simulink model "sysgenMRIDemo"  (Simulink 7.7)
settings: Solver=VariableStepDiscrete  StartTime=0.0  StopTime=inf  RelTol=1e-3
PreLoadFcn:
  | sysgenMRIDemo_PreloadFcn
InitFcn:
  | xlFrameDisplay;
undefined symbols (not defined in the file or in its folder): a, b, c_image_cols, c_image_rows, c_num_fstores, c_swathe_size, sysgenMRIDemo_data_imag_channel, xlFrameDisplay
libraries: xbsIndex_r4 x297, dspsrcs4 x3, xbsCopyrightNotice_r4 x1, simulink x1
(part 2 of 3)

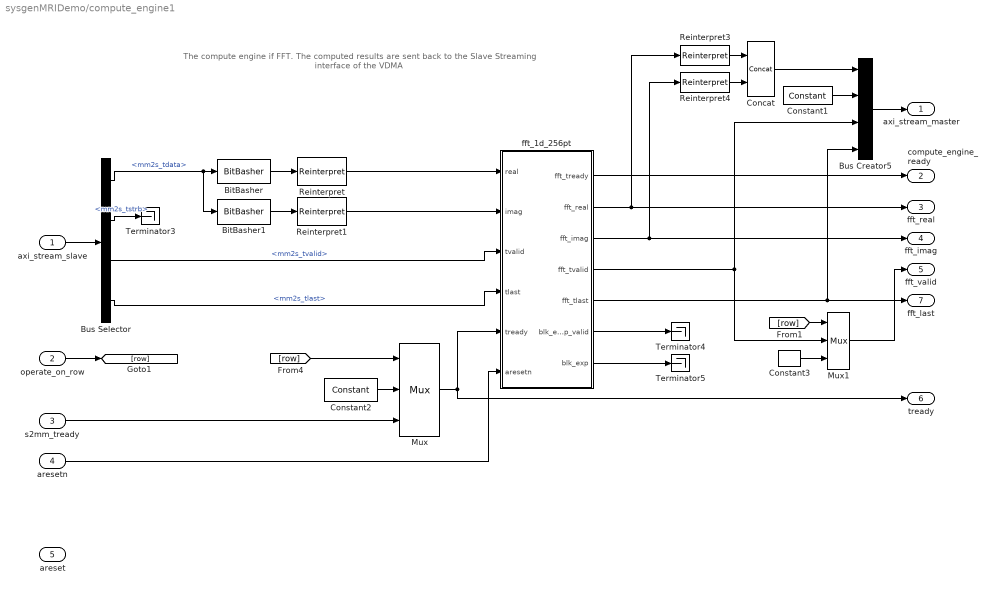
== system sysgenMRIDemo/compute_engine1 ==
  note: The compute engine if FFT. The computed results are sent back
      | to the Slave Streaming interface of the VDMA
  axi_stream_slave : Inport
  operate_on_row : Inport  Port=2
  s2mm_tready : Inport  Port=3
  aresetn : Inport  Port=4
  areset : Inport  Port=5
  BitBasher : xbsIndex_r4/BitBasher  bitexpr=|  display_expr=off  sr_1=1  arith_type1=Unsigned  bin_pt1=0  sr_2=2  arith_type2=Unsigned  bin_pt2=0  sr_3=3  arith_type3=Unsigned  bin_pt3=0  sr_4=4  arith_type4=Unsigned  bin_pt4=0  dbl_ovrd=off  block_type=bitbasher
      | <!DOCTYPE HTML PUBLIC "-//W3C//DTD HTML 4.0//EN" "http://www.w3.org/TR/REC-html40/strict.dtd">
      | <html><head><meta name="qrichtext" content="1" /><style type="text/css">
      | p, li { white-space: pre-wrap; }
      | </style></head><body style=" font-family:'MS Shell Dlg 2'; font-size:7.8pt; font-weight:400; font-style:normal;">
      | <p style=" margin-top:12px; margin-bottom:12px; margin-left:0px; margin-right:0px; -qt-block-indent:0; text-indent:0px;"><span style=" font-family:'MS Shell Dlg'; font-size:8pt;">real = {data[63:32]}</span></p></body></html>
      settings: block_version=12.3
  BitBasher1 : xbsIndex_r4/BitBasher  bitexpr=|  display_expr=off  sr_1=1  arith_type1=Unsigned  bin_pt1=0  sr_2=2  arith_type2=Unsigned  bin_pt2=0  sr_3=3  arith_type3=Unsigned  bin_pt3=0  sr_4=4  arith_type4=Unsigned  bin_pt4=0  dbl_ovrd=off  block_type=bitbasher
      | <!DOCTYPE HTML PUBLIC "-//W3C//DTD HTML 4.0//EN" "http://www.w3.org/TR/REC-html40/strict.dtd">
      | <html><head><meta name="qrichtext" content="1" /><style type="text/css">
      | p, li { white-space: pre-wrap; }
      | </style></head><body style=" font-family:'MS Shell Dlg 2'; font-size:7.8pt; font-weight:400; font-style:normal;">
      | <p style=" margin-top:12px; margin-bottom:12px; margin-left:0px; margin-right:0px; -qt-block-indent:0; text-indent:0px;"><span style=" font-family:'MS Shell Dlg'; font-size:8pt;">imag = {data[31:0]}</span></p></body></html>
      settings: block_version=12.3
  Bus Creator5 : BusCreator
  Bus Selector : BusSelector  OutputSignals=mm2s_tdata,mm2s_tstrb,mm2s_tvalid,mm2s_tlast
  Concat : xbsIndex_r4/Concat  num_inputs=2  dbl_ovrd=off  block_type=concat
      settings: block_version=12.3
  Constant1 : xbsIndex_r4/Constant  const=2^8-1  gui_display_data_type=Fixed-point  arith_type=Unsigned  n_bits=8  bin_pt=0  preci_type=Single  exp_width=8  frac_width=24  explicit_period=on  period=1  equ=P=C  opselect=C  inp2=PCIN>>17  opr=+  inp1=P  carry=CIN  dbl_ovrd=off  block_type=constant
      settings: block_version=12.3
  Constant2 : xbsIndex_r4/Constant  const=1  gui_display_data_type=Fixed-point  arith_type=Boolean  n_bits=8  bin_pt=0  preci_type=Single  exp_width=8  frac_width=24  explicit_period=on  period=1  equ=P=C  opselect=C  inp2=PCIN>>17  opr=+  inp1=P  carry=CIN  dbl_ovrd=off  block_type=constant
      settings: block_version=12.3
  Constant3 : xbsIndex_r4/Constant  const=0  gui_display_data_type=Fixed-point  arith_type=Boolean  n_bits=8  bin_pt=0  preci_type=Single  exp_width=8  frac_width=24  explicit_period=on  period=1  equ=P=C  opselect=C  inp2=PCIN>>17  opr=+  inp1=P  carry=CIN  dbl_ovrd=off  block_type=constant
      settings: block_version=12.3
  Mux : xbsIndex_r4/Mux  inputs=2  en=off  latency=0  precision=Full  arith_type=Unsigned  n_bits=16  bin_pt=14  quantization=Truncate  overflow=Wrap  dbl_ovrd=off  block_type=mux
      settings: block_version=13.0.2
  Mux1 : xbsIndex_r4/Mux  inputs=2  en=off  latency=0  precision=Full  arith_type=Unsigned  n_bits=16  bin_pt=14  quantization=Truncate  overflow=Wrap  dbl_ovrd=off  block_type=mux
      settings: block_version=13.0.2
  Reinterpret : xbsIndex_r4/Reinterpret  force_arith_type=on  arith_type="Signed  (2's comp)"  force_bin_pt=on  bin_pt=31  block_type=reinterpret
      settings: infoedit="Changes signal type without altering the binary representation.   You can changed the signal between signed and unsigned, and relocate the binary point.<br><br>Hardware notes: In hardware this block costs nothing.<br><br>Example:  Suppose the input is 6 bits wide, signed, with 2 fractional bits, and the output is forced to unsigned with 0 fractional bits.  Then an input of -2.0 (1110.00 in binary 2's complement) becomes an output of 56 (111000 in binary)."  block_version=12.3
  Reinterpret1 : xbsIndex_r4/Reinterpret  force_arith_type=on  arith_type="Signed  (2's comp)"  force_bin_pt=on  bin_pt=31  block_type=reinterpret
      settings: infoedit="Changes signal type without altering the binary representation.   You can changed the signal between signed and unsigned, and relocate the binary point.<br><br>Hardware notes: In hardware this block costs nothing.<br><br>Example:  Suppose the input is 6 bits wide, signed, with 2 fractional bits, and the output is forced to unsigned with 0 fractional bits.  Then an input of -2.0 (1110.00 in binary 2's complement) becomes an output of 56 (111000 in binary)."  block_version=12.3
  Reinterpret3 : xbsIndex_r4/Reinterpret  force_arith_type=on  arith_type=Unsigned  force_bin_pt=on  bin_pt=0  block_type=reinterpret
      settings: infoedit="Changes signal type without altering the binary representation.   You can changed the signal between signed and unsigned, and relocate the binary point.<br><br>Hardware notes: In hardware this block costs nothing.<br><br>Example:  Suppose the input is 6 bits wide, signed, with 2 fractional bits, and the output is forced to unsigned with 0 fractional bits.  Then an input of -2.0 (1110.00 in binary 2's complement) becomes an output of 56 (111000 in binary)."  block_version=12.3
  Reinterpret4 : xbsIndex_r4/Reinterpret  force_arith_type=on  arith_type=Unsigned  force_bin_pt=on  bin_pt=0  block_type=reinterpret
      settings: infoedit="Changes signal type without altering the binary representation.   You can changed the signal between signed and unsigned, and relocate the binary point.<br><br>Hardware notes: In hardware this block costs nothing.<br><br>Example:  Suppose the input is 6 bits wide, signed, with 2 fractional bits, and the output is forced to unsigned with 0 fractional bits.  Then an input of -2.0 (1110.00 in binary 2's complement) becomes an output of 56 (111000 in binary)."  block_version=12.3
  Terminator3 : Terminator
  Terminator4 : Terminator
  Terminator5 : Terminator
  fft_1d_256pt : Subsystem
  axi_stream_master : Outport
  compute_engine_ready : Outport  Port=2
  fft_real : Outport  Port=3
  fft_imag : Outport  Port=4
  fft_valid : Outport  Port=5
  tready : Outport  Port=6
  fft_last : Outport  Port=7
  wires:
  Reinterpret/1 -> fft_1d_256pt/1(real)
  BitBasher/1 -> Reinterpret/1
  BitBasher1/1 -> Reinterpret1/1
  Reinterpret1/1 -> fft_1d_256pt/2(imag)
  fft_1d_256pt/1(fft_tready) -> compute_engine_ready/1
  fft_1d_256pt/4(fft_tvalid) -> Bus Creator5/3, Mux1/2
  fft_1d_256pt/5(fft_tlast) -> fft_last/1, Bus Creator5/4
  fft_1d_256pt/2(fft_real) -> Reinterpret3/1, fft_real/1
  Reinterpret3/1 -> Concat/1
  Reinterpret4/1 -> Concat/2
  Concat/1 -> Bus Creator5/1
  Bus Selector/3 -> fft_1d_256pt/3(tvalid)  "<mm2s_tvalid>"
  fft_1d_256pt/3(fft_imag) -> Reinterpret4/1, fft_imag/1
  fft_1d_256pt/6(blk_exp_valid) -> Terminator4/1
  fft_1d_256pt/7(blk_exp) -> Terminator5/1
  axi_stream_slave/1 -> Bus Selector/1
  Bus Creator5/1 -> axi_stream_master/1
  Constant1/1 -> Bus Creator5/2
  Bus Selector/1 -> BitBasher/1, BitBasher1/1  "<mm2s_tdata>"
  Bus Selector/4 -> fft_1d_256pt/4(tlast)  "<mm2s_tlast>"
  Bus Selector/2 -> Terminator3/1  "<mm2s_tstrb>"
  Mux/1 -> fft_1d_256pt/5(tready), tready/1
  aresetn/1 -> fft_1d_256pt/6(aresetn)
  s2mm_tready/1 -> Mux/3
  [row] -> Mux/1
  operate_on_row/1 -> [row]
  Constant2/1 -> Mux/2
  [row] -> Mux1/1
  Mux1/1 -> fft_valid/1
  Constant3/1 -> Mux1/3

== system sysgenMRIDemo/data_collection ==
  In1 : Inport
  Enable : EnablePort
  Bus Creator1 : BusCreator  Inputs=3
  Bus to Vector : BusToVector
  Complex to Real-Imag : ComplexToRealImag
  Constant : Constant  Value=c_image_rows*c_image_cols-1
  Counter Free-Running : simulink/Sources/Counter Free-Running  SystemSampleTime=-1  NumBits=log2(c_image_rows*c_image_cols)  tsamp=1
  Data Type Conversion : DataTypeConversion  OutDataTypeStr=double
  Display : Display
  MATLAB Fcn : MATLABFcn  MATLABFcn=xlFrameDisplay(u(1),u(2),u(3), c_image_rows*c_image_cols)
  Relational Operator : RelationalOperator  Operator===  OutDataTypeStr=boolean
  Signal To Workspace : SignalToWorkspace  VariableName=mri_result_pl  SaveFormat=Array
      settings: CopyFcn=dspblkcopystw(gcbh);
  framesync : Outport
  wires:
  In1/1 -> Signal To Workspace/1, Complex to Real-Imag/1
  Counter Free-Running/1 -> Data Type Conversion/1
  Data Type Conversion/1 -> Relational Operator/1, Bus Creator1/1, Display/1
  Constant/1 -> Relational Operator/2
  Relational Operator/1 -> framesync/1
  Complex to Real-Imag/1 -> Bus Creator1/2
  Complex to Real-Imag/2 -> Bus Creator1/3
  Bus Creator1/1 -> Bus to Vector/1
  Bus to Vector/1 -> MATLAB Fcn/1

== system sysgenMRIDemo/image_Src1 ==
  next_data : Inport
  Subsystem : Subsystem
  Terminator : Terminator
  MRIReal : Outport
  MRIImag : Outport  Port=2
  wires:
  next_data/1 -> Subsystem/Enable
  Subsystem/1(MriReal) -> MRIReal/1
  Subsystem/2(MriImag) -> MRIImag/1
  Subsystem/3(MriDataValid) -> Terminator/1

== system sysgenMRIDemo/Data To AXI Streaming/EOF GEN ==
  In2 : Inport
  In1 : Inport  Port=2
  Counter : xbsIndex_r4/Counter  cnt_type=Count Limited  cnt_to=burst_length-1  operation=Up  start_count=0  cnt_by_val=1  arith_type=Unsigned  n_bits=ceil(log2(burst_length))+1  bin_pt=0  load_pin=off  rst=on  en=on  explicit_period=on  period=1  dbl_ovrd=off  use_behavioral_HDL=off  implementation=Fabric  block_type=counter
      settings: block_version=12.3
  Relational : xbsIndex_r4/Relational  mode=a=b  en=off  latency=0  dbl_ovrd=off  block_type=relational
      settings: block_version=12.3
  tvalid1 : xbsIndex_r4/Constant  const=burst_length-1  gui_display_data_type=Fixed-point  arith_type=Unsigned  n_bits=ceil(log2(burst_length))+1  bin_pt=0  preci_type=Single  exp_width=8  frac_width=24  explicit_period=on  period=1  equ=P=C  opselect=C  inp2=PCIN>>17  opr=+  inp1=P  carry=CIN  dbl_ovrd=off  block_type=constant
      settings: block_version=12.3
  Out1 : Outport
  wires:
  Counter/1 -> Relational/1  "data_count"
  tvalid1/1 -> Relational/2
  In1/1 -> Counter/1
  In2/1 -> Counter/2
  Relational/1 -> Out1/1

== system sysgenMRIDemo/Data To AXI Streaming/TLAST_GEN ==
  In2 : Inport
  In1 : Inport  Port=2
  Counter1 : xbsIndex_r4/Counter  cnt_type=Count Limited  cnt_to=c_image_cols-1  operation=Up  start_count=0  cnt_by_val=1  arith_type=Unsigned  n_bits=ceil(log2(c_image_cols))+1  bin_pt=0  load_pin=off  rst=on  en=on  explicit_period=on  period=1  dbl_ovrd=off  use_behavioral_HDL=off  implementation=Fabric  block_type=counter
      settings: block_version=12.3
  Relational1 : xbsIndex_r4/Relational  mode=a=b  en=off  latency=0  dbl_ovrd=off  block_type=relational
      settings: block_version=12.3
  tvalid3 : xbsIndex_r4/Constant  const=c_image_cols-1  gui_display_data_type=Fixed-point  arith_type=Unsigned  n_bits=ceil(log2(c_image_cols))+1  bin_pt=0  preci_type=Single  exp_width=8  frac_width=24  explicit_period=on  period=1  equ=P=C  opselect=C  inp2=PCIN>>17  opr=+  inp1=P  carry=CIN  dbl_ovrd=off  block_type=constant
      settings: block_version=12.3
  Out1 : Outport
  wires:
  Counter1/1 -> Relational1/1
  tvalid3/1 -> Relational1/2
  In1/1 -> Counter1/1
  In2/1 -> Counter1/2
  Relational1/1 -> Out1/1  "TLAST"

== system sysgenMRIDemo/Data To AXI Streaming/TVALID_GEN ==
  tvalid_in : Inport
  eof : Inport  Port=2
  txn : Inport  Port=3
  reset : Inport  Port=4
  Constant : xbsIndex_r4/Constant  const=1  gui_display_data_type=Fixed-point  arith_type=Boolean  n_bits=16  bin_pt=14  preci_type=Single  exp_width=8  frac_width=24  explicit_period=off  period=1  equ=P=C  opselect=C  inp2=PCIN>>17  opr=+  inp1=P  carry=CIN  dbl_ovrd=off  block_type=constant
      settings: block_version=13.0.2
  Constant1 : xbsIndex_r4/Constant  const=0  gui_display_data_type=Fixed-point  arith_type=Boolean  n_bits=16  bin_pt=14  preci_type=Single  exp_width=8  frac_width=24  explicit_period=off  period=1  equ=P=C  opselect=C  inp2=PCIN>>17  opr=+  inp1=P  carry=CIN  dbl_ovrd=off  block_type=constant
      settings: block_version=13.0.2
  Logical1 : xbsIndex_r4/Logical  logical_function=AND  inputs=2  en=off  latency=0  precision=Full  arith_type=Unsigned  n_bits=16  bin_pt=0  align_bp=on  dbl_ovrd=off  block_type=logical
      settings: block_version=12.3
  Mux : xbsIndex_r4/Mux  inputs=2  en=off  latency=0  precision=Full  arith_type=Unsigned  n_bits=16  bin_pt=14  quantization=Truncate  overflow=Wrap  dbl_ovrd=off  block_type=mux
      settings: block_version=13.0.2
  Register : xbsIndex_r4/Register  init=0  rst=on  en=on  dbl_ovrd=off  block_type=register
      settings: block_version=13.0.2
  tvalid_out : Outport
  wires:
  Constant/1 -> Register/1
  Register/1 -> Mux/1
  Constant1/1 -> Mux/3
  reset/1 -> Register/2
  tvalid_in/1 -> Mux/2
  Mux/1 -> tvalid_out/1
  Logical1/1 -> Register/3
  eof/1 -> Logical1/1
  txn/1 -> Logical1/2

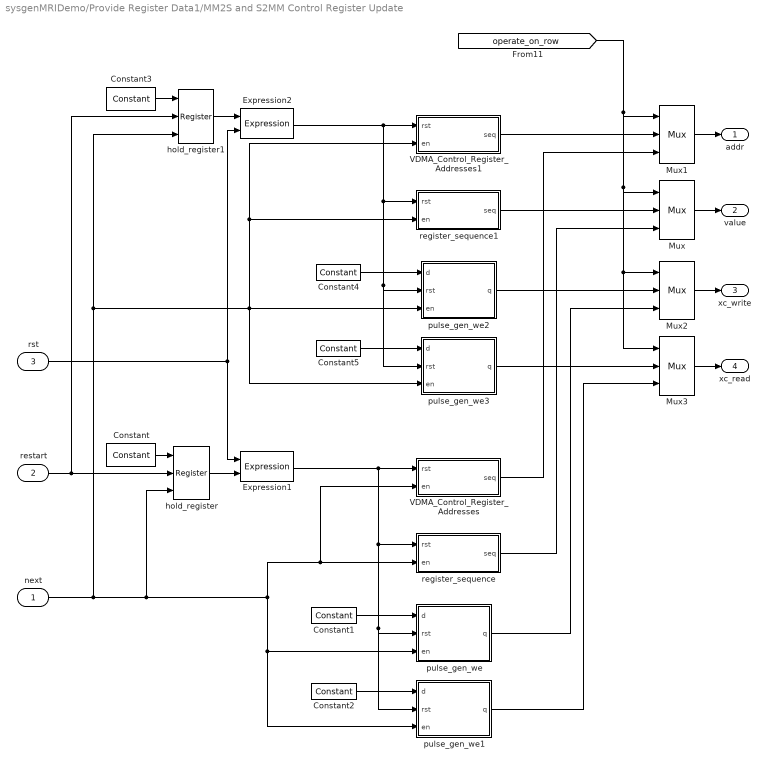
== system sysgenMRIDemo/Provide Register Data1/MM2S and S2MM Control Register Update ==
  next : Inport
  restart : Inport  Port=2
  rst : Inport  Port=3
  Constant : xbsIndex_r4/Constant  const=0  gui_display_data_type=Fixed-point  arith_type=Boolean  n_bits=16  bin_pt=14  preci_type=Single  exp_width=8  frac_width=24  explicit_period=off  period=1  equ=P=C  opselect=C  inp2=PCIN>>17  opr=+  inp1=P  carry=CIN  dbl_ovrd=off  block_type=constant
      settings: block_version=12.3
  Constant1 : xbsIndex_r4/Constant  const=0  gui_display_data_type=Fixed-point  arith_type=Boolean  n_bits=32  bin_pt=0  preci_type=Single  exp_width=8  frac_width=24  explicit_period=on  period=1  equ=P=C  opselect=C  inp2=PCIN>>17  opr=+  inp1=P  carry=CIN  dbl_ovrd=off  block_type=constant
      settings: block_version=12.3
  Constant2 : xbsIndex_r4/Constant  const=1  gui_display_data_type=Fixed-point  arith_type=Boolean  n_bits=32  bin_pt=0  preci_type=Single  exp_width=8  frac_width=24  explicit_period=on  period=1  equ=P=C  opselect=C  inp2=PCIN>>17  opr=+  inp1=P  carry=CIN  dbl_ovrd=off  block_type=constant
      settings: block_version=12.3
  Constant3 : xbsIndex_r4/Constant  const=0  gui_display_data_type=Fixed-point  arith_type=Boolean  n_bits=16  bin_pt=14  preci_type=Single  exp_width=8  frac_width=24  explicit_period=off  period=1  equ=P=C  opselect=C  inp2=PCIN>>17  opr=+  inp1=P  carry=CIN  dbl_ovrd=off  block_type=constant
      settings: block_version=12.3
  Constant4 : xbsIndex_r4/Constant  const=0  gui_display_data_type=Fixed-point  arith_type=Boolean  n_bits=32  bin_pt=0  preci_type=Single  exp_width=8  frac_width=24  explicit_period=on  period=1  equ=P=C  opselect=C  inp2=PCIN>>17  opr=+  inp1=P  carry=CIN  dbl_ovrd=off  block_type=constant
      settings: block_version=12.3
  Constant5 : xbsIndex_r4/Constant  const=1  gui_display_data_type=Fixed-point  arith_type=Boolean  n_bits=32  bin_pt=0  preci_type=Single  exp_width=8  frac_width=24  explicit_period=on  period=1  equ=P=C  opselect=C  inp2=PCIN>>17  opr=+  inp1=P  carry=CIN  dbl_ovrd=off  block_type=constant
      settings: block_version=12.3
  Expression1 : xbsIndex_r4/Expression  expression=a | b  align_bp=on  en=off  latency=0  precision=Full  arith_type=Unsigned  n_bits=16  bin_pt=0  dbl_ovrd=off  block_type=expr
      settings: block_version=12.3
  Expression2 : xbsIndex_r4/Expression  expression=a | b  align_bp=on  en=off  latency=0  precision=Full  arith_type=Unsigned  n_bits=16  bin_pt=0  dbl_ovrd=off  block_type=expr
      settings: block_version=12.3
  Mux{,1..3} (4 alike) : xbsIndex_r4/Mux  inputs=2  en=off  latency=0  precision=Full  arith_type=Unsigned  n_bits=16  bin_pt=14  quantization=Truncate  overflow=Wrap  dbl_ovrd=off  block_type=mux
      settings: block_version=13.0.2
  VDMA_Control_Register_Addresses : Subsystem  mask{c_sequence=[hex2dec('34') hex2dec('40') hex2dec('30') hex2dec('38') hex2dec('34') hex2dec('10') hex2dec('0') hex2dec('8') hex2dec('4')]}
      mask prompts: c_sequence "User sequence"
  VDMA_Control_Register_Addresses1 : Subsystem  mask{c_sequence=[hex2dec('4') hex2dec('10') hex2dec('0') hex2dec('8') hex2dec('4')]}
      mask prompts: c_sequence "User sequence"
  hold_register : xbsIndex_r4/Register  init=1  rst=on  en=on  dbl_ovrd=off  block_type=register
      settings: block_version=12.3
  hold_register1 : xbsIndex_r4/Register  init=1  rst=on  en=on  dbl_ovrd=off  block_type=register
      settings: block_version=12.3
  pulse_gen_we : Subsystem
  pulse_gen_we1 : Subsystem
  pulse_gen_we2 : Subsystem
  pulse_gen_we3 : Subsystem
  register_sequence : Subsystem  mask{c_sequence=[0 (1024+(min(c_num_frames_to_read,c_num_fstores)-1)*32) hex2dec(['00' dec2hex(min(c_num_frames_to_read,c_num_fstores),2) '1013']) 1024 hex2dec('00007000') (min(c_num_frames_to_read,c_num_fstores)-1)*32  hex2dec(['00' dec2hex(min(c_num_frames_to_read,c_num_fstores),2) '1013']) 0 hex2dec('00007000')]}
      mask prompts: c_sequence "User sequence"
  register_sequence1 : Subsystem  mask{c_sequence=[hex2dec('00007000') (min(c_num_frames_to_read,c_num_fstores)-1)*32  hex2dec(['00' dec2hex(min(c_num_frames_to_read,c_num_fstores),2) '1013']) 0 hex2dec('00007000')]}
      mask prompts: c_sequence "User sequence"
  addr : Outport
  value : Outport  Port=2
  xc_write : Outport  Port=3
  xc_read : Outport  Port=4
  wires:
  Constant2/1 -> pulse_gen_we1/1(d)
  restart/1 -> hold_register1/2, hold_register/2
  Constant/1 -> hold_register/1
  next/1 -> pulse_gen_we1/3(en), pulse_gen_we/3(en), register_sequence/2(en), VDMA_Control_Register_Addresses/2(en), hold_register/3, pulse_gen_we3/3(en), pulse_gen_we2/3(en), register_sequence1/2(en), VDMA_Control_Register_Addresses1/2(en), hold_register1/3
  Expression1/1 -> VDMA_Control_Register_Addresses/1(rst), pulse_gen_we1/2(rst), pulse_gen_we/2(rst), register_sequence/1(rst)
  VDMA_Control_Register_Addresses/1(seq) -> Mux1/3
  register_sequence/1(seq) -> Mux/3
  pulse_gen_we/1(q) -> Mux2/3
  Constant1/1 -> pulse_gen_we/1(d)
  pulse_gen_we1/1(q) -> Mux3/3
  Constant5/1 -> pulse_gen_we3/1(d)
  Constant3/1 -> hold_register1/1
  Expression2/1 -> VDMA_Control_Register_Addresses1/1(rst), pulse_gen_we3/2(rst), pulse_gen_we2/2(rst), register_sequence1/1(rst)
  VDMA_Control_Register_Addresses1/1(seq) -> Mux1/2
  register_sequence1/1(seq) -> Mux/2
  pulse_gen_we2/1(q) -> Mux2/2
  Constant4/1 -> pulse_gen_we2/1(d)
  pulse_gen_we3/1(q) -> Mux3/2
  Mux1/1 -> addr/1
  Mux/1 -> value/1
  Mux2/1 -> xc_write/1
  Mux3/1 -> xc_read/1
  [operate_on_row] -> Mux1/1, Mux/1, Mux2/1, Mux3/1
  hold_register1/1 -> Expression2/1
  rst/1 -> Expression2/2, Expression1/1
  hold_register/1 -> Expression1/2

== system sysgenMRIDemo/Provide Register Data1/S2MM Control Register Update ==
  next : Inport
  restart : Inport  Port=2
  rst : Inport  Port=3
  Constant : xbsIndex_r4/Constant  const=0  gui_display_data_type=Fixed-point  arith_type=Boolean  n_bits=16  bin_pt=14  preci_type=Single  exp_width=8  frac_width=24  explicit_period=off  period=1  equ=P=C  opselect=C  inp2=PCIN>>17  opr=+  inp1=P  carry=CIN  dbl_ovrd=off  block_type=constant
      settings: block_version=12.3
  Constant1 : xbsIndex_r4/Constant  const=0  gui_display_data_type=Fixed-point  arith_type=Boolean  n_bits=32  bin_pt=0  preci_type=Single  exp_width=8  frac_width=24  explicit_period=on  period=1  equ=P=C  opselect=C  inp2=PCIN>>17  opr=+  inp1=P  carry=CIN  dbl_ovrd=off  block_type=constant
      settings: block_version=12.3
  Constant2 : xbsIndex_r4/Constant  const=1  gui_display_data_type=Fixed-point  arith_type=Boolean  n_bits=32  bin_pt=0  preci_type=Single  exp_width=8  frac_width=24  explicit_period=on  period=1  equ=P=C  opselect=C  inp2=PCIN>>17  opr=+  inp1=P  carry=CIN  dbl_ovrd=off  block_type=constant
      settings: block_version=12.3
  Expression1 : xbsIndex_r4/Expression  expression=a | b  align_bp=on  en=off  latency=0  precision=Full  arith_type=Unsigned  n_bits=16  bin_pt=0  dbl_ovrd=off  block_type=expr
      settings: block_version=12.3
  VDMA_Control_Register_Addresses : Subsystem  mask{c_sequence=[hex2dec('34') hex2dec('40') hex2dec('30') hex2dec('38') hex2dec('34')]}
      mask prompts: c_sequence "User sequence"
  VDMA_Control_Register_Data2 : Subsystem  mask{c_sequence=[hex2dec('00007000') (min(c_num_frames_to_write,c_num_fstores)-1)*32 hex2dec(['00' dec2hex(min(c_num_frames_to_write,c_num_fstores),2) '1013']) 0 hex2dec('00007000')]}
      mask prompts: c_sequence "User sequence"
  hold_register : xbsIndex_r4/Register  init=1  rst=on  en=on  dbl_ovrd=off  block_type=register
      settings: block_version=12.3
  pulse_gen_re : Subsystem
  pulse_gen_we : Subsystem
  addr : Outport
  value : Outport  Port=2
  xc_write : Outport  Port=3
  xc_read : Outport  Port=4
  wires:
  restart/1 -> hold_register/2
  Constant/1 -> hold_register/1
  Expression1/1 -> pulse_gen_re/2(rst), pulse_gen_we/2(rst), VDMA_Control_Register_Data2/1(rst), VDMA_Control_Register_Addresses/1(rst)
  pulse_gen_re/1(q) -> xc_read/1
  Constant2/1 -> pulse_gen_re/1(d)
  Constant1/1 -> pulse_gen_we/1(d)
  pulse_gen_we/1(q) -> xc_write/1
  VDMA_Control_Register_Data2/1(seq) -> value/1
  VDMA_Control_Register_Addresses/1(seq) -> addr/1
  next/1 -> pulse_gen_re/3(en), pulse_gen_we/3(en), VDMA_Control_Register_Addresses/2(en), VDMA_Control_Register_Data2/2(en), hold_register/3
  hold_register/1 -> Expression1/1
  rst/1 -> Expression1/2

== system sysgenMRIDemo/Provide Register Data1/change_detectpor ==
  in : Inport
  rst : Inport  Port=2
  Constant : xbsIndex_r4/Constant  const=0  gui_display_data_type=Fixed-point  arith_type=Unsigned  n_bits=1  bin_pt=0  preci_type=Single  exp_width=8  frac_width=24  explicit_period=off  period=1  equ=P=C  opselect=C  inp2=PCIN>>17  opr=+  inp1=P  carry=CIN  dbl_ovrd=off  block_type=constant
      settings: block_version=12.3
  Logical : xbsIndex_r4/Logical  logical_function=XOR  inputs=2  en=off  latency=0  precision=Full  arith_type=Unsigned  n_bits=16  bin_pt=0  align_bp=on  dbl_ovrd=off  block_type=logical
      settings: block_version=12.3
  Register1 : xbsIndex_r4/Register  init=0  rst=on  en=off  dbl_ovrd=off  block_type=register
      settings: block_version=12.3
  Relational : xbsIndex_r4/Relational  mode=a!=b  en=off  latency=0  dbl_ovrd=off  block_type=relational
      settings: block_version=12.3
  change : Outport
  wires:
  Register1/1 -> Logical/2
  in/1 -> Register1/1, Logical/1
  Logical/1 -> Relational/1
  Constant/1 -> Relational/2
  Relational/1 -> change/1
  rst/1 -> Register1/2

== system sysgenMRIDemo/Provide Register Data1/change_detectpor1 ==
  in : Inport
  rst : Inport  Port=2
  Constant : xbsIndex_r4/Constant  const=0  gui_display_data_type=Fixed-point  arith_type=Unsigned  n_bits=1  bin_pt=0  preci_type=Single  exp_width=8  frac_width=24  explicit_period=off  period=1  equ=P=C  opselect=C  inp2=PCIN>>17  opr=+  inp1=P  carry=CIN  dbl_ovrd=off  block_type=constant
      settings: block_version=12.3
  Logical : xbsIndex_r4/Logical  logical_function=XOR  inputs=2  en=off  latency=0  precision=Full  arith_type=Unsigned  n_bits=16  bin_pt=0  align_bp=on  dbl_ovrd=off  block_type=logical
      settings: block_version=12.3
  Register1 : xbsIndex_r4/Register  init=0  rst=on  en=off  dbl_ovrd=off  block_type=register
      settings: block_version=12.3
  Relational : xbsIndex_r4/Relational  mode=a!=b  en=off  latency=0  dbl_ovrd=off  block_type=relational
      settings: block_version=12.3
  change : Outport
  wires:
  Register1/1 -> Logical/2
  in/1 -> Register1/1, Logical/1
  Logical/1 -> Relational/1
  Constant/1 -> Relational/2
  Relational/1 -> change/1
  rst/1 -> Register1/2

== system sysgenMRIDemo/Provide Register Data1/count_down ==
  rst : Inport
  en : Inport  Port=2
  Constant3 : xbsIndex_r4/Constant  const=0  gui_display_data_type=Fixed-point  arith_type=Unsigned  n_bits=ceil(ceil( (c_image_rows/c_swathe_size) / c_num_fstores) + 1)  bin_pt=0  preci_type=Single  exp_width=8  frac_width=24  explicit_period=off  period=1  equ=P=C  opselect=C  inp2=PCIN>>17  opr=+  inp1=P  carry=CIN  dbl_ovrd=off  block_type=constant
      settings: block_version=12.3
  Counter : xbsIndex_r4/Counter  cnt_type=Count Limited  cnt_to=0  operation=Down  start_count=init_val  cnt_by_val=1  arith_type=Unsigned  n_bits=ceil(log2(init_val + 1))  bin_pt=0  load_pin=off  rst=on  en=on  explicit_period=on  period=1  dbl_ovrd=off  use_behavioral_HDL=off  implementation=Fabric  block_type=counter
      settings: block_version=12.3
  Expression : xbsIndex_r4/Expression  expression=a & b  align_bp=on  en=off  latency=0  precision=Full  arith_type=Unsigned  n_bits=16  bin_pt=0  dbl_ovrd=off  block_type=expr
      settings: block_version=12.3
  Relational1 : xbsIndex_r4/Relational  mode=a!=b  en=off  latency=0  dbl_ovrd=off  block_type=relational
      settings: block_version=12.3
  cnt : Outport
  wires:
  en/1 -> Expression/2
  Relational1/1 -> Expression/1
  Constant3/1 -> Relational1/2
  Counter/1 -> cnt/1, Relational1/1
  Expression/1 -> Counter/2
  rst/1 -> Counter/1

== system sysgenMRIDemo/Provide Register Data1/count_down1 ==
  rst : Inport
  en : Inport  Port=2
  Constant3 : xbsIndex_r4/Constant  const=0  gui_display_data_type=Fixed-point  arith_type=Unsigned  n_bits=ceil(ceil( (c_image_rows/c_swathe_size) / c_num_fstores) + 1)  bin_pt=0  preci_type=Single  exp_width=8  frac_width=24  explicit_period=off  period=1  equ=P=C  opselect=C  inp2=PCIN>>17  opr=+  inp1=P  carry=CIN  dbl_ovrd=off  block_type=constant
      settings: block_version=12.3
  Counter : xbsIndex_r4/Counter  cnt_type=Count Limited  cnt_to=0  operation=Down  start_count=init_val  cnt_by_val=1  arith_type=Unsigned  n_bits=ceil(log2(init_val + 1))  bin_pt=0  load_pin=off  rst=on  en=on  explicit_period=on  period=1  dbl_ovrd=off  use_behavioral_HDL=off  implementation=Fabric  block_type=counter
      settings: block_version=12.3
  Expression : xbsIndex_r4/Expression  expression=a & b  align_bp=on  en=off  latency=0  precision=Full  arith_type=Unsigned  n_bits=16  bin_pt=0  dbl_ovrd=off  block_type=expr
      settings: block_version=12.3
  Relational1 : xbsIndex_r4/Relational  mode=a!=b  en=off  latency=0  dbl_ovrd=off  block_type=relational
      settings: block_version=12.3
  cnt : Outport
  wires:
  en/1 -> Expression/2
  Relational1/1 -> Expression/1
  Constant3/1 -> Relational1/2
  Counter/1 -> cnt/1, Relational1/1
  Expression/1 -> Counter/2
  rst/1 -> Counter/1

== system sysgenMRIDemo/Provide Register Data1/is_zero ==
  in : Inport
  Constant4 : xbsIndex_r4/Constant  const=0  gui_display_data_type=Fixed-point  arith_type=Unsigned  n_bits=1  bin_pt=0  preci_type=Single  exp_width=8  frac_width=24  explicit_period=off  period=1  equ=P=C  opselect=C  inp2=PCIN>>17  opr=+  inp1=P  carry=CIN  dbl_ovrd=off  block_type=constant
      settings: block_version=12.3
  Relational1 : xbsIndex_r4/Relational  mode=a=b  en=off  latency=0  dbl_ovrd=off  block_type=relational
      settings: block_version=12.3
  out : Outport
  wires:
  Constant4/1 -> Relational1/2
  in/1 -> Relational1/1
  Relational1/1 -> out/1

== system sysgenMRIDemo/Provide Register Data1/is_zero1 ==
  in : Inport
  Constant4 : xbsIndex_r4/Constant  const=0  gui_display_data_type=Fixed-point  arith_type=Unsigned  n_bits=1  bin_pt=0  preci_type=Single  exp_width=8  frac_width=24  explicit_period=off  period=1  equ=P=C  opselect=C  inp2=PCIN>>17  opr=+  inp1=P  carry=CIN  dbl_ovrd=off  block_type=constant
      settings: block_version=12.3
  Relational1 : xbsIndex_r4/Relational  mode=a=b  en=off  latency=0  dbl_ovrd=off  block_type=relational
      settings: block_version=12.3
  out : Outport
  wires:
  Constant4/1 -> Relational1/2
  in/1 -> Relational1/1
  Relational1/1 -> out/1

== system sysgenMRIDemo/Provide Register Data1/rising_edge_detector ==
  in : Inport
  rst : Inport  Port=2
  Expression : xbsIndex_r4/Expression  expression=a & ~b  align_bp=on  en=off  latency=0  precision=Full  arith_type=Unsigned  n_bits=16  bin_pt=0  dbl_ovrd=off  block_type=expr
      settings: block_version=12.3
  Register1 : xbsIndex_r4/Register  init=0  rst=on  en=off  dbl_ovrd=off  block_type=register
      settings: block_version=12.3
  rise : Outport
  wires:
  Expression/1 -> rise/1
  in/1 -> Register1/1, Expression/1
  Register1/1 -> Expression/2
  rst/1 -> Register1/2

== system sysgenMRIDemo/Provide Register Data1/rising_edge_detector1 ==
  in : Inport
  rst : Inport  Port=2
  Expression : xbsIndex_r4/Expression  expression=a & ~b  align_bp=on  en=off  latency=0  precision=Full  arith_type=Unsigned  n_bits=16  bin_pt=0  dbl_ovrd=off  block_type=expr
      settings: block_version=12.3
  Register1 : xbsIndex_r4/Register  init=0  rst=on  en=off  dbl_ovrd=off  block_type=register
      settings: block_version=12.3
  rise : Outport
  wires:
  Expression/1 -> rise/1
  in/1 -> Register1/1, Expression/1
  Register1/1 -> Expression/2
  rst/1 -> Register1/2

== system sysgenMRIDemo/Provide Register Data1/zero_router ==
  sel : Inport
  i : Inport  Port=2
  Expression : xbsIndex_r4/Expression  expression=a ^ b  align_bp=on  en=off  latency=0  precision=Full  arith_type=Unsigned  n_bits=16  bin_pt=0  dbl_ovrd=off  block_type=expr
      settings: block_version=12.3
  Mux : xbsIndex_r4/Mux  inputs=2  en=off  latency=0  precision=Full  arith_type=Unsigned  n_bits=16  bin_pt=14  quantization=Truncate  overflow=Wrap  dbl_ovrd=off  block_type=mux
      settings: block_version=12.3
  Mux1 : xbsIndex_r4/Mux  inputs=2  en=off  latency=0  precision=Full  arith_type=Unsigned  n_bits=16  bin_pt=14  quantization=Truncate  overflow=Wrap  dbl_ovrd=off  block_type=mux
      settings: block_version=12.3
  o0 : Outport
  o1 : Outport  Port=2
  wires:
  Expression/1 -> Mux/3, Mux1/2
  sel/1 -> Mux/1, Mux1/1
  i/1 -> Mux/2, Expression/1, Expression/2, Mux1/3
  Mux/1 -> o0/1
  Mux1/1 -> o1/1

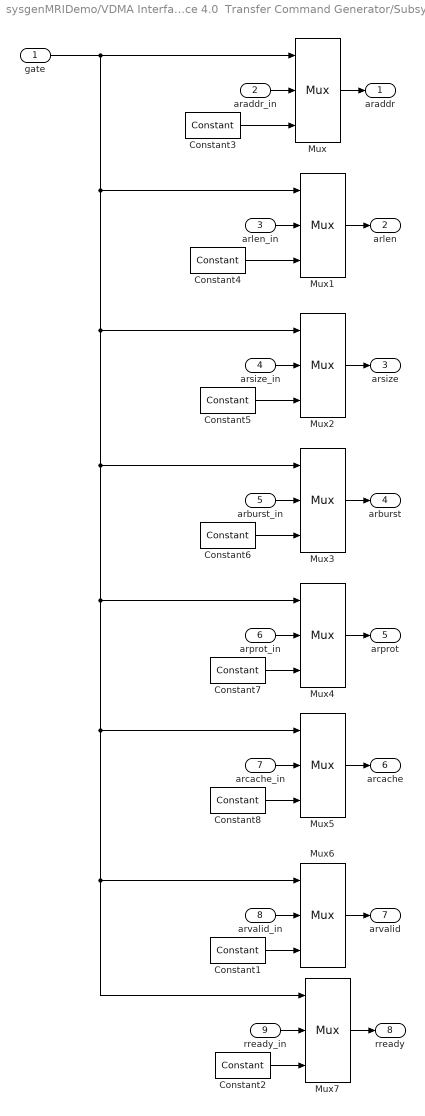
== system sysgenMRIDemo/VDMA Interface 4.0  Transfer Command Generator/Subsystem ==
  gate : Inport
  araddr_in : Inport  Port=2
  arlen_in : Inport  Port=3
  arsize_in : Inport  Port=4
  arburst_in : Inport  Port=5
  arprot_in : Inport  Port=6
  arcache_in : Inport  Port=7
  arvalid_in : Inport  Port=8
  rready_in : Inport  Port=9
  Constant1 : xbsIndex_r4/Constant  const=0  gui_display_data_type=Fixed-point  arith_type=Boolean  n_bits=4  bin_pt=0  preci_type=Single  exp_width=8  frac_width=24  explicit_period=off  period=1  equ=P=C  opselect=C  inp2=PCIN>>17  opr=+  inp1=P  carry=CIN  dbl_ovrd=off  block_type=constant
      settings: block_version=12.3
  Constant2 : xbsIndex_r4/Constant  const=0  gui_display_data_type=Fixed-point  arith_type=Boolean  n_bits=4  bin_pt=0  preci_type=Single  exp_width=8  frac_width=24  explicit_period=off  period=1  equ=P=C  opselect=C  inp2=PCIN>>17  opr=+  inp1=P  carry=CIN  dbl_ovrd=off  block_type=constant
      settings: block_version=12.3
  Constant3 : xbsIndex_r4/Constant  const=0  gui_display_data_type=Fixed-point  arith_type=Unsigned  n_bits=32  bin_pt=0  preci_type=Single  exp_width=8  frac_width=24  explicit_period=off  period=1  equ=P=C  opselect=C  inp2=PCIN>>17  opr=+  inp1=P  carry=CIN  dbl_ovrd=off  block_type=constant
      settings: block_version=12.3
  Constant4 : xbsIndex_r4/Constant  const=0  gui_display_data_type=Fixed-point  arith_type=Unsigned  n_bits=8  bin_pt=0  preci_type=Single  exp_width=8  frac_width=24  explicit_period=off  period=1  equ=P=C  opselect=C  inp2=PCIN>>17  opr=+  inp1=P  carry=CIN  dbl_ovrd=off  block_type=constant
      settings: block_version=12.3
  Constant5 : xbsIndex_r4/Constant  const=0  gui_display_data_type=Fixed-point  arith_type=Unsigned  n_bits=3  bin_pt=0  preci_type=Single  exp_width=8  frac_width=24  explicit_period=off  period=1  equ=P=C  opselect=C  inp2=PCIN>>17  opr=+  inp1=P  carry=CIN  dbl_ovrd=off  block_type=constant
      settings: block_version=12.3
  Constant6 : xbsIndex_r4/Constant  const=0  gui_display_data_type=Fixed-point  arith_type=Unsigned  n_bits=2  bin_pt=0  preci_type=Single  exp_width=8  frac_width=24  explicit_period=off  period=1  equ=P=C  opselect=C  inp2=PCIN>>17  opr=+  inp1=P  carry=CIN  dbl_ovrd=off  block_type=constant
      settings: block_version=12.3
  Constant7 : xbsIndex_r4/Constant  const=0  gui_display_data_type=Fixed-point  arith_type=Unsigned  n_bits=3  bin_pt=0  preci_type=Single  exp_width=8  frac_width=24  explicit_period=off  period=1  equ=P=C  opselect=C  inp2=PCIN>>17  opr=+  inp1=P  carry=CIN  dbl_ovrd=off  block_type=constant
      settings: block_version=12.3
  Constant8 : xbsIndex_r4/Constant  const=0  gui_display_data_type=Fixed-point  arith_type=Unsigned  n_bits=4  bin_pt=0  preci_type=Single  exp_width=8  frac_width=24  explicit_period=off  period=1  equ=P=C  opselect=C  inp2=PCIN>>17  opr=+  inp1=P  carry=CIN  dbl_ovrd=off  block_type=constant
      settings: block_version=12.3
  Mux{,1..7} (8 alike) : xbsIndex_r4/Mux  inputs=2  en=off  latency=0  precision=Full  arith_type=Unsigned  n_bits=16  bin_pt=14  quantization=Truncate  overflow=Wrap  dbl_ovrd=off  block_type=mux
      settings: block_version=12.3
  araddr : Outport
  arlen : Outport  Port=2
  arsize : Outport  Port=3
  arburst : Outport  Port=4
  arprot : Outport  Port=5
  arcache : Outport  Port=6
  arvalid : Outport  Port=7
  rready : Outport  Port=8
  wires:
  Mux7/1 -> rready/1
  rready_in/1 -> Mux7/2
  Constant2/1 -> Mux7/3
  Mux6/1 -> arvalid/1
  arvalid_in/1 -> Mux6/2
  Constant1/1 -> Mux6/3
  Mux5/1 -> arcache/1
  arcache_in/1 -> Mux5/2
  Mux4/1 -> arprot/1
  arprot_in/1 -> Mux4/2
  Mux3/1 -> arburst/1
  arburst_in/1 -> Mux3/2
  Mux2/1 -> arsize/1
  arsize_in/1 -> Mux2/2
  Mux1/1 -> arlen/1
  arlen_in/1 -> Mux1/2
  Mux/1 -> araddr/1
  araddr_in/1 -> Mux/2
  gate/1 -> Mux7/1, Mux6/1, Mux5/1, Mux4/1, Mux3/1, Mux2/1, Mux1/1, Mux/1
  Constant8/1 -> Mux5/3
  Constant7/1 -> Mux4/3
  Constant6/1 -> Mux3/3
  Constant5/1 -> Mux2/3
  Constant4/1 -> Mux1/3
  Constant3/1 -> Mux/3

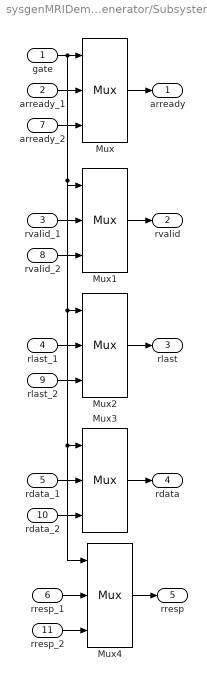
== system sysgenMRIDemo/VDMA Interface 4.0  Transfer Command Generator/Subsystem1 ==
  gate : Inport
  arready_1 : Inport  Port=2
  rvalid_1 : Inport  Port=3
  rlast_1 : Inport  Port=4
  rdata_1 : Inport  Port=5
  rresp_1 : Inport  Port=6
  arready_2 : Inport  Port=7
  rvalid_2 : Inport  Port=8
  rlast_2 : Inport  Port=9
  rdata_2 : Inport  Port=10
  rresp_2 : Inport  Port=11
  Mux{,1..4} (5 alike) : xbsIndex_r4/Mux  inputs=2  en=off  latency=0  precision=Full  arith_type=Unsigned  n_bits=16  bin_pt=14  quantization=Truncate  overflow=Wrap  dbl_ovrd=off  block_type=mux
      settings: block_version=12.3
  arready : Outport
  rvalid : Outport  Port=2
  rlast : Outport  Port=3
  rdata : Outport  Port=4
  rresp : Outport  Port=5
  wires:
  rresp_2/1 -> Mux4/3
  Mux4/1 -> rresp/1
  rresp_1/1 -> Mux4/2
  rdata_2/1 -> Mux3/3
  Mux3/1 -> rdata/1
  rdata_1/1 -> Mux3/2
  rlast_2/1 -> Mux2/3
  Mux2/1 -> rlast/1
  rlast_1/1 -> Mux2/2
  rvalid_2/1 -> Mux1/3
  Mux1/1 -> rvalid/1
  rvalid_1/1 -> Mux1/2
  arready_2/1 -> Mux/3
  Mux/1 -> arready/1
  arready_1/1 -> Mux/2
  gate/1 -> Mux4/1, Mux3/1, Mux2/1, Mux1/1, Mux/1

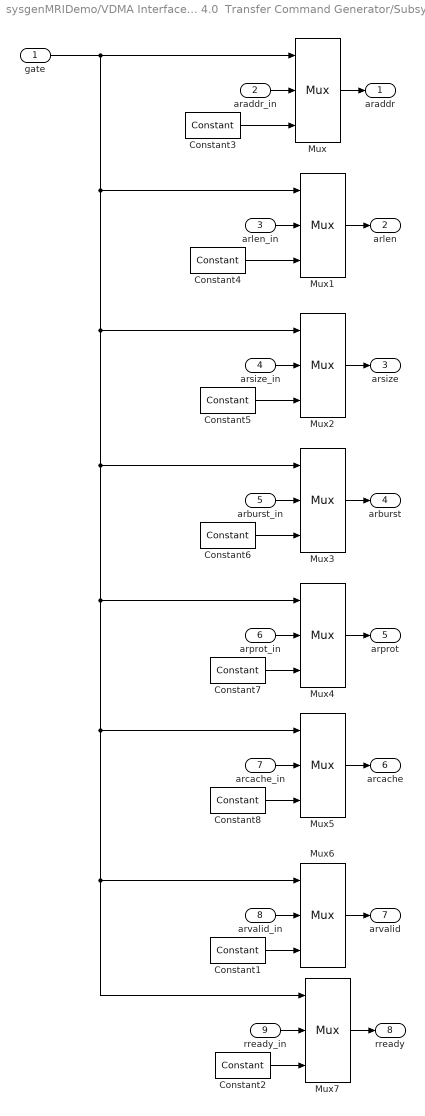
== system sysgenMRIDemo/VDMA Interface 4.0  Transfer Command Generator/Subsystem4 ==
  gate : Inport
  araddr_in : Inport  Port=2
  arlen_in : Inport  Port=3
  arsize_in : Inport  Port=4
  arburst_in : Inport  Port=5
  arprot_in : Inport  Port=6
  arcache_in : Inport  Port=7
  arvalid_in : Inport  Port=8
  rready_in : Inport  Port=9
  Constant1 : xbsIndex_r4/Constant  const=0  gui_display_data_type=Fixed-point  arith_type=Boolean  n_bits=4  bin_pt=0  preci_type=Single  exp_width=8  frac_width=24  explicit_period=off  period=1  equ=P=C  opselect=C  inp2=PCIN>>17  opr=+  inp1=P  carry=CIN  dbl_ovrd=off  block_type=constant
      settings: block_version=12.3
  Constant2 : xbsIndex_r4/Constant  const=0  gui_display_data_type=Fixed-point  arith_type=Boolean  n_bits=4  bin_pt=0  preci_type=Single  exp_width=8  frac_width=24  explicit_period=off  period=1  equ=P=C  opselect=C  inp2=PCIN>>17  opr=+  inp1=P  carry=CIN  dbl_ovrd=off  block_type=constant
      settings: block_version=12.3
  Constant3 : xbsIndex_r4/Constant  const=0  gui_display_data_type=Fixed-point  arith_type=Unsigned  n_bits=32  bin_pt=0  preci_type=Single  exp_width=8  frac_width=24  explicit_period=off  period=1  equ=P=C  opselect=C  inp2=PCIN>>17  opr=+  inp1=P  carry=CIN  dbl_ovrd=off  block_type=constant
      settings: block_version=12.3
  Constant4 : xbsIndex_r4/Constant  const=0  gui_display_data_type=Fixed-point  arith_type=Unsigned  n_bits=8  bin_pt=0  preci_type=Single  exp_width=8  frac_width=24  explicit_period=off  period=1  equ=P=C  opselect=C  inp2=PCIN>>17  opr=+  inp1=P  carry=CIN  dbl_ovrd=off  block_type=constant
      settings: block_version=12.3
  Constant5 : xbsIndex_r4/Constant  const=0  gui_display_data_type=Fixed-point  arith_type=Unsigned  n_bits=3  bin_pt=0  preci_type=Single  exp_width=8  frac_width=24  explicit_period=off  period=1  equ=P=C  opselect=C  inp2=PCIN>>17  opr=+  inp1=P  carry=CIN  dbl_ovrd=off  block_type=constant
      settings: block_version=12.3
  Constant6 : xbsIndex_r4/Constant  const=0  gui_display_data_type=Fixed-point  arith_type=Unsigned  n_bits=2  bin_pt=0  preci_type=Single  exp_width=8  frac_width=24  explicit_period=off  period=1  equ=P=C  opselect=C  inp2=PCIN>>17  opr=+  inp1=P  carry=CIN  dbl_ovrd=off  block_type=constant
      settings: block_version=12.3
  Constant7 : xbsIndex_r4/Constant  const=0  gui_display_data_type=Fixed-point  arith_type=Unsigned  n_bits=3  bin_pt=0  preci_type=Single  exp_width=8  frac_width=24  explicit_period=off  period=1  equ=P=C  opselect=C  inp2=PCIN>>17  opr=+  inp1=P  carry=CIN  dbl_ovrd=off  block_type=constant
      settings: block_version=12.3
  Constant8 : xbsIndex_r4/Constant  const=0  gui_display_data_type=Fixed-point  arith_type=Unsigned  n_bits=4  bin_pt=0  preci_type=Single  exp_width=8  frac_width=24  explicit_period=off  period=1  equ=P=C  opselect=C  inp2=PCIN>>17  opr=+  inp1=P  carry=CIN  dbl_ovrd=off  block_type=constant
      settings: block_version=12.3
  Mux{,1..7} (8 alike) : xbsIndex_r4/Mux  inputs=2  en=off  latency=0  precision=Full  arith_type=Unsigned  n_bits=16  bin_pt=14  quantization=Truncate  overflow=Wrap  dbl_ovrd=off  block_type=mux
      settings: block_version=12.3
  araddr : Outport
  arlen : Outport  Port=2
  arsize : Outport  Port=3
  arburst : Outport  Port=4
  arprot : Outport  Port=5
  arcache : Outport  Port=6
  arvalid : Outport  Port=7
  rready : Outport  Port=8
  wires:
  Constant3/1 -> Mux/3
  Constant4/1 -> Mux1/3
  Constant5/1 -> Mux2/3
  Constant6/1 -> Mux3/3
  Constant7/1 -> Mux4/3
  Constant8/1 -> Mux5/3
  gate/1 -> Mux/1, Mux1/1, Mux2/1, Mux3/1, Mux4/1, Mux5/1, Mux6/1, Mux7/1
  araddr_in/1 -> Mux/2
  Mux/1 -> araddr/1
  arlen_in/1 -> Mux1/2
  Mux1/1 -> arlen/1
  arsize_in/1 -> Mux2/2
  Mux2/1 -> arsize/1
  arburst_in/1 -> Mux3/2
  Mux3/1 -> arburst/1
  arprot_in/1 -> Mux4/2
  Mux4/1 -> arprot/1
  arcache_in/1 -> Mux5/2
  Mux5/1 -> arcache/1
  Constant1/1 -> Mux6/3
  arvalid_in/1 -> Mux6/2
  Mux6/1 -> arvalid/1
  Constant2/1 -> Mux7/3
  rready_in/1 -> Mux7/2
  Mux7/1 -> rready/1

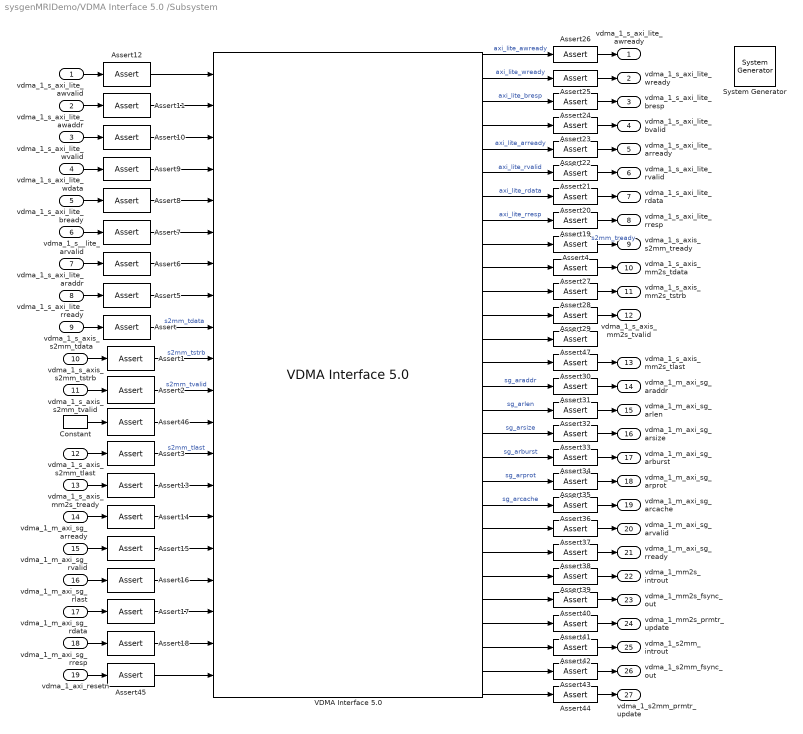
== system sysgenMRIDemo/VDMA Interface 5.0 /Subsystem ==
  vdma_1_s_axi_lite_awvalid : Inport
  vdma_1_s_axi_lite_awaddr : Inport  Port=2
  vdma_1_s_axi_lite_wvalid : Inport  Port=3
  vdma_1_s_axi_lite_wdata : Inport  Port=4
  vdma_1_s_axi_lite_bready : Inport  Port=5
  vdma_1_s__lite_arvalid : Inport  Port=6
  vdma_1_s_axi_lite_araddr : Inport  Port=7
  vdma_1_s_axi_lite_rready : Inport  Port=8
  vdma_1_s_axis_s2mm_tdata : Inport  Port=9
  vdma_1_s_axis_s2mm_tstrb : Inport  Port=10
  vdma_1_s_axis_s2mm_tvalid : Inport  Port=11
  vdma_1_s_axis_s2mm_tlast : Inport  Port=12
  vdma_1_s_axis_mm2s_tready : Inport  Port=13
  vdma_1_m_axi_sg_arready : Inport  Port=14
  vdma_1_m_axi_sg_rvalid : Inport  Port=15
  vdma_1_m_axi_sg_rlast : Inport  Port=16
  vdma_1_m_axi_sg_rdata : Inport  Port=17
  vdma_1_m_axi_sg_rresp : Inport  Port=18
  vdma_1_axi_resetn : Inport  Port=19
  " System Generator" : xbsIndex_r4/ System Generator  Tag=genX  SystemSampleTime=-1  xilinxfamily=virtex6  part=xc6vlx240t  speed=-1  package=ff1156  synthesis_tool=XST  clock_wrapper=Clock Enables  directory=./netlist  proj_type=Project Navigator  Synth_file=XST Defaults  Impl_file=ISE Defaults  testbench=off  simulink_period=1  sysclk_period=20  dcm_input_clock_period=10  incr_netlist=off  trim_vbits=Everywhere in SubSystem  dbl_ovrd=According to Block Masks  core_generation=According to Block Masks  run_coregen=off  deprecated_control=off  eval_field=0  block_type=sysgen
      settings: block_version=12.3
  Assert{,1..47} (48 alike) : xbsIndex_r4/Assert  assert_type=off  type_source=Explicitly  gui_display_data_type=Fixed-point  arith_type="Signed  (2's comp)"  n_bits=16  bin_pt=14  preci_type=Single  exp_width=8  frac_width=24  assert_rate=off  rate_source=Explicitly  period=1  output_port=on  block_type=assert
      settings: block_version=12.3
  Constant : xbsIndex_r4/Constant  const=1  gui_display_data_type=Fixed-point  arith_type=Unsigned  n_bits=1  bin_pt=0  preci_type=Single  exp_width=8  frac_width=24  explicit_period=on  period=1  equ=P=C  opselect=C  inp2=PCIN>>17  opr=+  inp1=P  carry=CIN  dbl_ovrd=off  block_type=constant
  "VDMA Interface 5.0 " : xbsIndex_r4/VDMA Interface 5.0   c_mem_size=64MB  c_number_of_vdma_if=1  c_stream_if_configuration_1=Master/Slave  c_no_of_frames_1=c_num_fstores  c_use_fsync_1=off  c_flush_on_fsync_1=off  c_use_sg_engine_1=on  c_video_prm_read_1=on  c_m_axis_mm2s_data_width_1=64  c_m_axis_mm2s_frame_sync_tuser_1=off  c_mm2s_linebuffer_depth_1=0  c_mm2s_linebuffer_threshold_1=1  c_s_axis_s2mm_data_width_1=64  c_s_axis_s2mm_frame_sync_tuser_1=off  c_s2mm_linebuffer_depth_1=0  c_s2mm_linebuffer_threshold_1=1  c_stream_if_configuration_2=Master/Slave  c_no_of_frames_2=3  c_use_fsync_2=off  c_flush_on_fsync_2=off  c_use_sg_engine_2=off  c_video_prm_read_2=on  c_m_axis_mm2s_data_width_2=32  c_m_axis_mm2s_frame_sync_tuser_2=off  c_mm2s_linebuffer_depth_2=0  c_mm2s_linebuffer_threshold_2=1  c_s_axis_s2mm_data_width_2=32  c_s_axis_s2mm_frame_sync_tuser_2=off  c_s2mm_linebuffer_depth_2=0  c_s2mm_linebuffer_threshold_2=1  c_stream_if_configuration_3=Master/Slave  c_no_of_frames_3=3  c_use_fsync_3=off  c_flush_on_fsync_3=off  c_use_sg_engine_3=off  c_video_prm_read_3=on  c_m_axis_mm2s_data_width_3=32  c_m_axis_mm2s_frame_sync_tuser_3=off  c_mm2s_linebuffer_depth_3=0  c_mm2s_linebuffer_threshold_3=1  c_s_axis_s2mm_data_width_3=32  c_s_axis_s2mm_frame_sync_tuser_3=off  c_s2mm_linebuffer_depth_3=0  c_s2mm_linebuffer_threshold_3=1  c_stream_if_configuration_4=Master/Slave  c_no_of_frames_4=3  c_use_fsync_4=off  c_flush_on_fsync_4=off  c_use_sg_engine_4=off  c_video_prm_read_4=on  c_m_axis_mm2s_data_width_4=32  c_m_axis_mm2s_frame_sync_tuser_4=off  c_mm2s_linebuffer_depth_4=0  c_mm2s_linebuffer_threshold_4=1  c_s_axis_s2mm_data_width_4=32  c_s_axis_s2mm_frame_sync_tuser_4=off  c_s2mm_linebuffer_depth_4=0  c_s2mm_linebuffer_threshold_4=1  simulation_model='emi_v5_0:EMI_v5_0_Model'  block_type=vdma
      settings: infoedit="This is a bit-accurate simulation model for multiple AXI VDMA external memory interfaces.  Netlisting will generate the port interface that can be attached to the VDMA IP.  This block is currently in beta."
  vdma_1_s_axi_lite_awready : Outport
  vdma_1_s_axi_lite_wready : Outport  Port=2
  vdma_1_s_axi_lite_bresp : Outport  Port=3
  vdma_1_s_axi_lite_bvalid : Outport  Port=4
  vdma_1_s_axi_lite_arready : Outport  Port=5
  vdma_1_s_axi_lite_rvalid : Outport  Port=6
  vdma_1_s_axi_lite_rdata : Outport  Port=7
  vdma_1_s_axi_lite_rresp : Outport  Port=8
  vdma_1_s_axis_s2mm_tready : Outport  Port=9
  vdma_1_s_axis_mm2s_tdata : Outport  Port=10
  vdma_1_s_axis_mm2s_tstrb : Outport  Port=11
  vdma_1_s_axis_mm2s_tvalid : Outport  Port=12
  vdma_1_s_axis_mm2s_tlast : Outport  Port=13
  vdma_1_m_axi_sg_araddr : Outport  Port=14
  vdma_1_m_axi_sg_arlen : Outport  Port=15
  vdma_1_m_axi_sg_arsize : Outport  Port=16
  vdma_1_m_axi_sg_arburst : Outport  Port=17
  vdma_1_m_axi_sg_arprot : Outport  Port=18
  vdma_1_m_axi_sg_arcache : Outport  Port=19
  vdma_1_m_axi_sg_arvalid : Outport  Port=20
  vdma_1_m_axi_sg_rready : Outport  Port=21
  vdma_1_mm2s_introut : Outport  Port=22
  vdma_1_mm2s_fsync_out : Outport  Port=23
  vdma_1_mm2s_prmtr_update : Outport  Port=24
  vdma_1_s2mm_introut : Outport  Port=25
  vdma_1_s2mm_fsync_out : Outport  Port=26
  vdma_1_s2mm_prmtr_update : Outport  Port=27
  wires:
  "VDMA Interface 5.0 "/10 -> Assert27/1
  "VDMA Interface 5.0 "/11 -> Assert28/1
  "VDMA Interface 5.0 "/12 -> Assert29/1
  "VDMA Interface 5.0 "/14 -> Assert30/1
  Assert/1 -> "VDMA Interface 5.0 "/9  "s2mm_tdata"
  Assert1/1 -> "VDMA Interface 5.0 "/10  "s2mm_tstrb"
  Assert2/1 -> "VDMA Interface 5.0 "/11  "s2mm_tvalid"
  Assert3/1 -> "VDMA Interface 5.0 "/13  "s2mm_tlast"
  Assert5/1 -> "VDMA Interface 5.0 "/8
  Assert6/1 -> "VDMA Interface 5.0 "/7
  Assert7/1 -> "VDMA Interface 5.0 "/6
  Assert8/1 -> "VDMA Interface 5.0 "/5
  Assert9/1 -> "VDMA Interface 5.0 "/4
  Assert10/1 -> "VDMA Interface 5.0 "/3
  Assert11/1 -> "VDMA Interface 5.0 "/2
  Assert12/1 -> "VDMA Interface 5.0 "/1
  Assert13/1 -> "VDMA Interface 5.0 "/14
  Assert14/1 -> "VDMA Interface 5.0 "/15
  Assert15/1 -> "VDMA Interface 5.0 "/16
  "VDMA Interface 5.0 "/1 -> Assert26/1  "axi_lite_awready"
  "VDMA Interface 5.0 "/2 -> Assert25/1  "axi_lite_wready"
  "VDMA Interface 5.0 "/3 -> Assert24/1  "axi_lite_bresp"
  "VDMA Interface 5.0 "/5 -> Assert22/1  "axi_lite_arready"
  "VDMA Interface 5.0 "/6 -> Assert21/1  "axi_lite_rvalid"
  "VDMA Interface 5.0 "/7 -> Assert20/1  "axi_lite_rdata"
  "VDMA Interface 5.0 "/8 -> Assert19/1  "axi_lite_rresp"
  Assert45/1 -> "VDMA Interface 5.0 "/20
  vdma_1_s_axi_lite_awvalid/1 -> Assert12/1
  Assert26/1 -> vdma_1_s_axi_lite_awready/1
  vdma_1_s_axi_lite_awaddr/1 -> Assert11/1
  Assert25/1 -> vdma_1_s_axi_lite_wready/1
  vdma_1_s_axi_lite_wvalid/1 -> Assert10/1
  Assert24/1 -> vdma_1_s_axi_lite_bresp/1
  Assert23/1 -> vdma_1_s_axi_lite_bvalid/1
  vdma_1_s_axi_lite_wdata/1 -> Assert9/1
  Assert22/1 -> vdma_1_s_axi_lite_arready/1
  Assert21/1 -> vdma_1_s_axi_lite_rvalid/1
  vdma_1_s_axi_lite_bready/1 -> Assert8/1
  Assert20/1 -> vdma_1_s_axi_lite_rdata/1
  vdma_1_s__lite_arvalid/1 -> Assert7/1
  Assert19/1 -> vdma_1_s_axi_lite_rresp/1
  Assert4/1 -> vdma_1_s_axis_s2mm_tready/1  "s2mm_tready"
  vdma_1_s_axi_lite_araddr/1 -> Assert6/1
  Assert27/1 -> vdma_1_s_axis_mm2s_tdata/1
  vdma_1_s_axi_lite_rready/1 -> Assert5/1
  Assert28/1 -> vdma_1_s_axis_mm2s_tstrb/1
  Assert29/1 -> vdma_1_s_axis_mm2s_tvalid/1
  vdma_1_s_axis_s2mm_tdata/1 -> Assert/1
  Assert30/1 -> vdma_1_s_axis_mm2s_tlast/1
  vdma_1_s_axis_s2mm_tstrb/1 -> Assert1/1
  Assert31/1 -> vdma_1_m_axi_sg_araddr/1
  Assert32/1 -> vdma_1_m_axi_sg_arlen/1
  vdma_1_s_axis_s2mm_tvalid/1 -> Assert2/1
  Assert33/1 -> vdma_1_m_axi_sg_arsize/1
  Assert34/1 -> vdma_1_m_axi_sg_arburst/1
  vdma_1_s_axis_s2mm_tlast/1 -> Assert3/1
  Assert35/1 -> vdma_1_m_axi_sg_arprot/1
  vdma_1_s_axis_mm2s_tready/1 -> Assert13/1
  Assert36/1 -> vdma_1_m_axi_sg_arcache/1
  Assert37/1 -> vdma_1_m_axi_sg_arvalid/1
  vdma_1_m_axi_sg_arready/1 -> Assert14/1
  Assert38/1 -> vdma_1_m_axi_sg_rready/1
  vdma_1_m_axi_sg_rvalid/1 -> Assert15/1
  Assert39/1 -> vdma_1_mm2s_introut/1
  Assert40/1 -> vdma_1_mm2s_fsync_out/1
  vdma_1_m_axi_sg_rlast/1 -> Assert16/1
  Assert41/1 -> vdma_1_mm2s_prmtr_update/1
  Assert42/1 -> vdma_1_s2mm_introut/1
  vdma_1_m_axi_sg_rdata/1 -> Assert17/1
  Assert43/1 -> vdma_1_s2mm_fsync_out/1
  vdma_1_m_axi_sg_rresp/1 -> Assert18/1
  Assert44/1 -> vdma_1_s2mm_prmtr_update/1
  vdma_1_axi_resetn/1 -> Assert45/1
  Assert46/1 -> "VDMA Interface 5.0 "/12
  Assert16/1 -> "VDMA Interface 5.0 "/17
  Assert17/1 -> "VDMA Interface 5.0 "/18
  Assert18/1 -> "VDMA Interface 5.0 "/19
  "VDMA Interface 5.0 "/4 -> Assert23/1
  "VDMA Interface 5.0 "/9 -> Assert4/1
  "VDMA Interface 5.0 "/13 -> Assert47/1
  "VDMA Interface 5.0 "/15 -> Assert31/1  "sg_araddr"
  "VDMA Interface 5.0 "/16 -> Assert32/1  "sg_arlen"
  "VDMA Interface 5.0 "/17 -> Assert33/1  "sg_arsize"
  "VDMA Interface 5.0 "/18 -> Assert34/1  "sg_arburst"
  "VDMA Interface 5.0 "/19 -> Assert35/1  "sg_arprot"
  "VDMA Interface 5.0 "/20 -> Assert36/1  "sg_arcache"
  "VDMA Interface 5.0 "/21 -> Assert37/1
  "VDMA Interface 5.0 "/22 -> Assert38/1
  "VDMA Interface 5.0 "/23 -> Assert39/1
  "VDMA Interface 5.0 "/24 -> Assert40/1
  "VDMA Interface 5.0 "/25 -> Assert41/1
  "VDMA Interface 5.0 "/26 -> Assert42/1
  "VDMA Interface 5.0 "/27 -> Assert43/1
  "VDMA Interface 5.0 "/28 -> Assert44/1
  Constant/1 -> Assert46/1
